simulink model "instalatie_fara_filtru"  (R2022b)
settings: Solver=VariableStepAuto  StartTime=0.0  StopTime=10.0  RelTol=1e-3
values from neighbouring files (symbols this model uses):
  k = 0.035    [date_indrumator.m]    (also in proiect.m)
  k11 = k2^2 + 4*(k - k3)*k1    (= 0.08909684)    [date_indrumator.m]    (also in proiect.m = 0.08885985)
  k12 = 8*(k-k3)    (= 0.2848)    [date_indrumator.m]    (also in proiect.m)
  k13 = 2*(k-k3)    (= 0.0712)    [date_indrumator.m]    (also in proiect.m)
  k2 = -0.015    [date_indrumator.m]    (also in proiect.m = -0.0015)
  keta = 8*(10^-5)    (= 8e-05)    [date_indrumator.m]    (also in proiect.m)
settings Model: Creator=Ruxandra  LastModifiedBy=Ruxandra

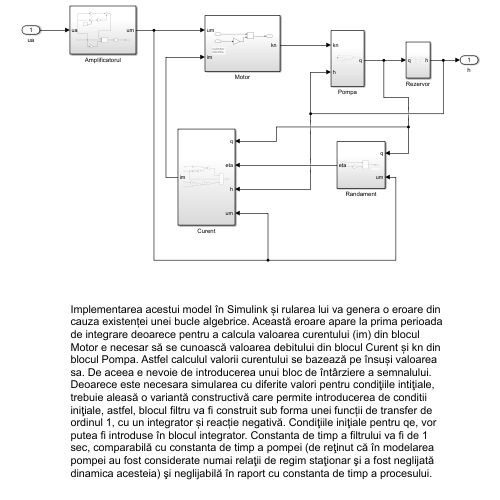
[thumbnail: Simulink's stored preview of the top-level diagram]
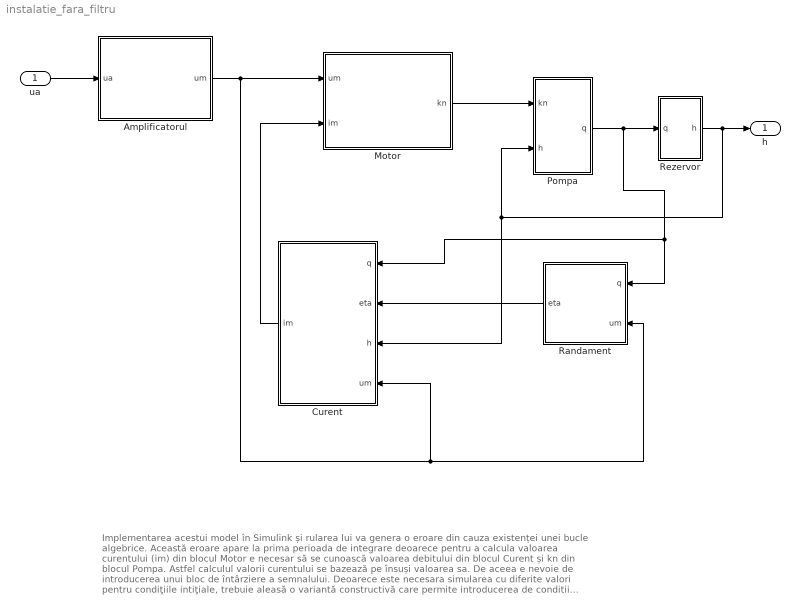
== system instalatie_fara_filtru ==
  note: Implementarea acestui model în Simulink și rularea lui va genera o eroare din cauza existenței unei bucle algebrice. Această eroare apare la prima perioada de integrare deoarece pentru a calcula valoarea curentului (im) din blocul Motor e necesar să se cunoască valoarea debitului din blocul Curent și kn din blocul Pompa. Astfel calculul valorii curentului se bazează pe însuși valoarea sa. De aceea e nevoie de introducerea unui bloc de întârziere a semnalului. Deoarece este necesara simularea cu diferite valori pentru condiţiile intiţiale, trebuie aleasă o variantă constructivă care permite introducerea de conditii iniţiale, astfel, blocul filtru va fi construit sub forma unei funcții de transfer de ordinul 1, cu un integrator și reacție negativă. Condiţiile iniţiale pentru qe, vor putea fi introduse în blocul integrator. Constanta de timp a filtrului va fi de 1 sec, comparabilă cu constanta de timp a pompei (de reţinut că în modelarea pompei au fost considerate numai relaţii de regim staţionar şi a fost neglijată dinamica acesteia) şi neglijabilă în raport cu constanta de timp a procesului.
  ua : Inport
  Amplificatorul : Subsystem
  Curent : Subsystem
  Motor : Subsystem
  Pompa : Subsystem
  Randament : Subsystem
  Rezervor : Subsystem
  h : Outport
  wires:
  ua/1 -> Amplificatorul/1(ua)
  Amplificatorul/1(um) -> Motor/1(um), Curent/4(um), Randament/2(um)
  Curent/1(im) -> Motor/2(im)
  Motor/1("kn ") -> Pompa/1(kn)
  Rezervor/1(h) -> Pompa/2(h), Curent/3(h), h/1
  Pompa/1(q) -> Curent/1(q), Randament/1(q), Rezervor/1(q)
  Randament/1(eta) -> Curent/2(eta)

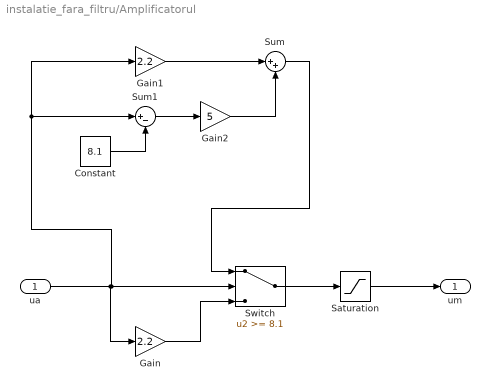
== system instalatie_fara_filtru/Amplificatorul ==
  ua : Inport
  Constant : Constant  Value=8.1
  Gain : Gain  Gain=2.2
  Gain1 : Gain  Gain=2.2
  Gain2 : Gain  Gain=5
  Saturation : Saturate  UpperLimit=22  LowerLimit=0
  Sum : Sum  Inputs=|++
  Sum1 : Sum  Inputs=|+-
  Switch : Switch  Threshold=8.1  RndMeth=Nearest  SaturateOnIntegerOverflow=off  InputSameDT=off
  um : Outport
  wires:
  Gain1/1 -> Sum/1
  ua/1 -> Sum1/1, Gain1/1, Switch/2, Gain/1
  Saturation/1 -> um/1
  Gain/1 -> Switch/3
  Gain2/1 -> Sum/2
  Sum1/1 -> Gain2/1
  Sum/1 -> Switch/1
  Switch/1 -> Saturation/1
  Constant/1 -> Sum1/2

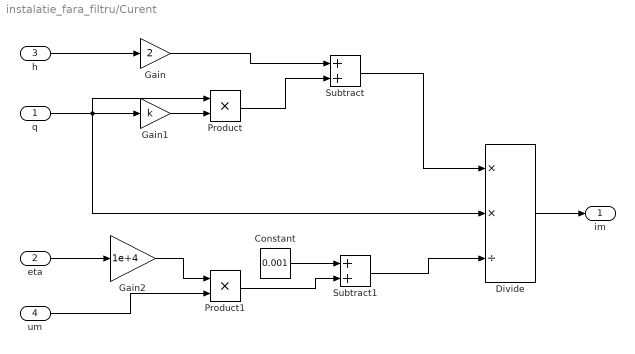
== system instalatie_fara_filtru/Curent ==
  q : Inport
  eta : Inport  Port=2
  h : Inport  Port=3
  um : Inport  Port=4
  Constant : Constant  Value=0.001
  Divide : Product  Inputs=**/
  Gain : Gain  Gain=2
  Gain1 : Gain  Gain=k
  Gain2 : Gain  Gain=1e+4
  Product : Product
  Product1 : Product
  Subtract : Sum
  Subtract1 : Sum
  im : Outport
  wires:
  Product/1 -> Subtract/2
  h/1 -> Gain/1
  Gain/1 -> Subtract/1
  Subtract1/1 -> Divide/3
  Gain2/1 -> Product1/1
  Constant/1 -> Subtract1/1
  Subtract/1 -> Divide/1
  Gain1/1 -> Product/2
  eta/1 -> Gain2/1
  Product1/1 -> Subtract1/2
  q/1 -> Divide/2, Gain1/1, Product/1
  um/1 -> Product1/2
  Divide/1 -> im/1

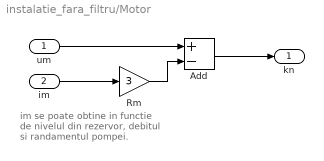
== system instalatie_fara_filtru/Motor ==
  note: im se poate obtine in functie de nivelul din rezervor, debitul si randamentul pompei.
  um : Inport
  im : Inport  Port=2
  Add : Sum  Inputs=+-
  Rm : Gain  Gain=3
  "kn " : Outport
  wires:
  im/1 -> Rm/1
  um/1 -> Add/1
  Rm/1 -> Add/2
  Add/1 -> "kn "/1

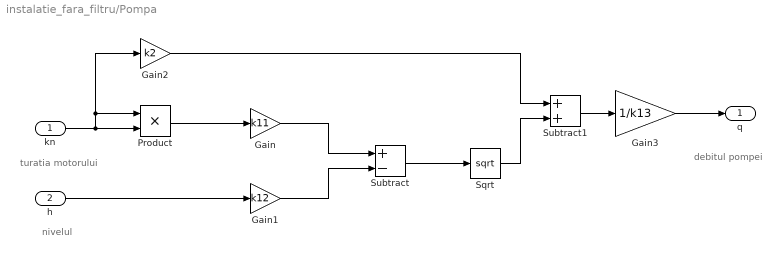
== system instalatie_fara_filtru/Pompa ==
  note: debitul pompei
  note: nivelul
  note: turatia motorului
  kn : Inport
  h : Inport  Port=2
  Gain : Gain  Gain=k11
  Gain1 : Gain  Gain=k12
  Gain2 : Gain  Gain=k2
  Gain3 : Gain  Gain=1/k13
  Product : Product
  Sqrt : Sqrt
  Subtract : Sum  Inputs=+-
  Subtract1 : Sum
  q : Outport
  wires:
  Sqrt/1 -> Subtract1/2
  Gain1/1 -> Subtract/2
  h/1 -> Gain1/1
  Gain2/1 -> Subtract1/1
  kn/1 -> Product/1, Gain2/1, Product/2
  Subtract/1 -> Sqrt/1
  Subtract1/1 -> Gain3/1
  Gain/1 -> Subtract/1
  Gain3/1 -> q/1
  Product/1 -> Gain/1

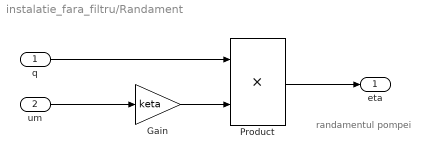
== system instalatie_fara_filtru/Randament ==
  note: randamentul pompei
  q : Inport
  um : Inport  Port=2
  Gain : Gain  Gain=keta
  Product : Product
  eta : Outport
  wires:
  um/1 -> Gain/1
  Product/1 -> eta/1
  q/1 -> Product/1
  Gain/1 -> Product/2

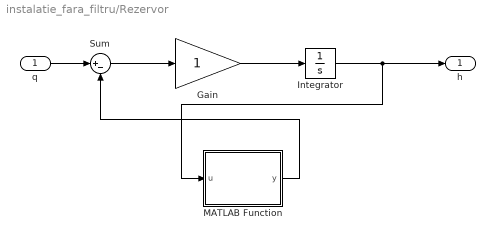
== system instalatie_fara_filtru/Rezervor ==
  q : Inport
  Gain : Gain
  Integrator : Integrator
  MATLAB Function : MATLAB Function  TreatAsAtomicUnit=on
  Sum : Sum  Inputs=|+-
  h : Outport
  wires:
  Integrator/1 -> h/1, MATLAB Function/1(u)
  q/1 -> Sum/1
  Gain/1 -> Integrator/1
  MATLAB Function/1(y) -> Sum/2
  Sum/1 -> Gain/1

== matlab function instalatie_fara_filtru/Rezervor/MATLAB Function ==
  data: u input; y output
function y = sqrt(u)

y = sqrt(u)*9;
